simulink model "open_model_with_delay"  (R2021b)
settings: Solver=FixedStepAuto  StartTime=0.0  StopTime=5000  FixedStep=0.005  RelTol=1e-3
settings Model: Creator=den  LastModifiedBy=den

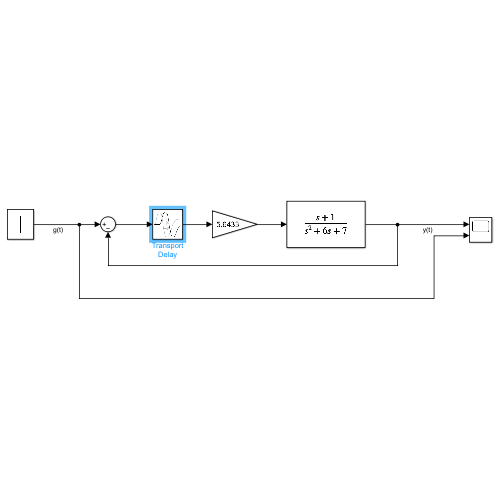
[thumbnail: Simulink's stored preview of the top-level diagram]
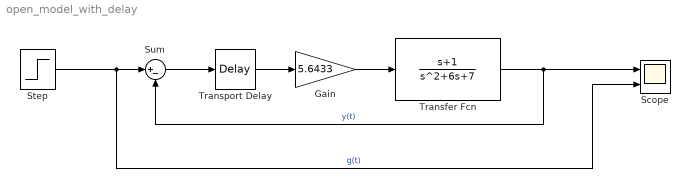
== system open_model_with_delay ==
  Gain : Gain  Gain=5.6433
  Scope : Scope  NumInputPorts=2
  Step : Step  SampleTime=0
  Sum : Sum  Inputs=|+-
  Transfer Fcn : TransferFcn  Numerator=[1 1]  Denominator=[1 6 7]
  Transport Delay : TransportDelay  DelayTime=5
  wires:
  Gain/1 -> Transfer Fcn/1
  Transport Delay/1 -> Gain/1
  Sum/1 -> Transport Delay/1
  Step/1 -> Scope/2, Sum/1  "g(t)"
  Transfer Fcn/1 -> Scope/1, Sum/2  "y(t)"
